simulink model "get_rho"  (R2017a)
settings: Solver=ode4  StartTime=0.0  StopTime=dT  FixedStep=dT  MaxStep=dT  RelTol=1e-3
undefined symbols (not defined in the file or in its folder): alt_init
libraries: atmospheric_library x1
settings Model: SimulationMode=accelerator  Creator=jack.marriott  LastModifiedBy=marriott
settings DataIOCC: SaveFormat=Array  ReturnWorkspaceOutputs=on  ReturnWorkspaceOutputsName=ksim
settings DebuggingCC: ReadBeforeWriteMsg=DisableAll  WriteAfterWriteMsg=DisableAll  WriteAfterReadMsg=DisableAll  MultiTaskDSMMsg=none
settings ModelReferenceCC: UpdateModelReferenceTargets=IfOutOfDate
settings SFSimCC: SFSimEcho=off

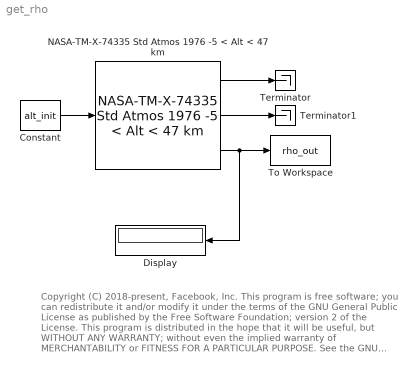
== system get_rho ==
  note: Copyright (C) 2018-present, Facebook, Inc.
      |
      | This program is free software; you can redistribute it and/or modify
      | it under the terms of the GNU General Public License as published by
      | the Free Software Foundation; version 2 of the License.
      |
      | This program is distributed in the hope that it will be useful,
      | but WITHOUT ANY WARRANTY; without even the implied warranty of
      | MERCHANTABILITY or FITNESS FOR A PARTICULAR PURPOSE. See the
      | GNU General Public License for more details.
      |
      | You should have received a copy of the GNU General Public License along
      | with this program; if not, write to the Free Software Foundation, Inc.,
      | 51 Franklin Street, Fifth Floor, Boston, MA 02110-1301 USA.
  Constant : Constant  Value=alt_init
  Display : Display
  NASA-TM-X-74335 Std Atmos 1976 -5 < Alt < 47 km : atmospheric_library/NASA-TM-X-74335 Std Atmos 1976 -5 < Alt < 47 km
  Terminator : Terminator
  Terminator1 : Terminator
  To Workspace : ToWorkspace  VariableName=rho_out  SaveFormat=Structure  SampleTime=-1
  wires:
  NASA-TM-X-74335 Std Atmos 1976 -5 < Alt < 47 km/1 -> Terminator/1
  NASA-TM-X-74335 Std Atmos 1976 -5 < Alt < 47 km/2 -> Terminator1/1
  NASA-TM-X-74335 Std Atmos 1976 -5 < Alt < 47 km/3 -> To Workspace/1, Display/1
  Constant/1 -> NASA-TM-X-74335 Std Atmos 1976 -5 < Alt < 47 km/1
